simulink model "esp_env"  (R2020b)
settings: Solver=VariableStepAuto  StartTime=0.0  StopTime=7.1  RelTol=1e-3
values from neighbouring files (symbols this model uses):
  Ts = 1.0    (= 1)    [demo_rl.m]
undefined symbols (not defined in the file or in its folder): A, B, C, D, K, L, steeringAngle
libraries: simulink x2
settings Model: Creator=Shreyash  LastModifiedBy=Asus
settings DataIOCC: ReturnWorkspaceOutputs=off
settings DebuggingCC: ArithmeticOperatorsInVariantConditions=warning
settings SFSimCC: SimUseLocalCustomCode=off  CustomCodeUndefinedFunction=UseInterfaceOnly
settings RTWCC: RTWUseLocalCustomCode=off

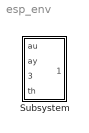
== system esp_env ==
  Subsystem : Subsystem

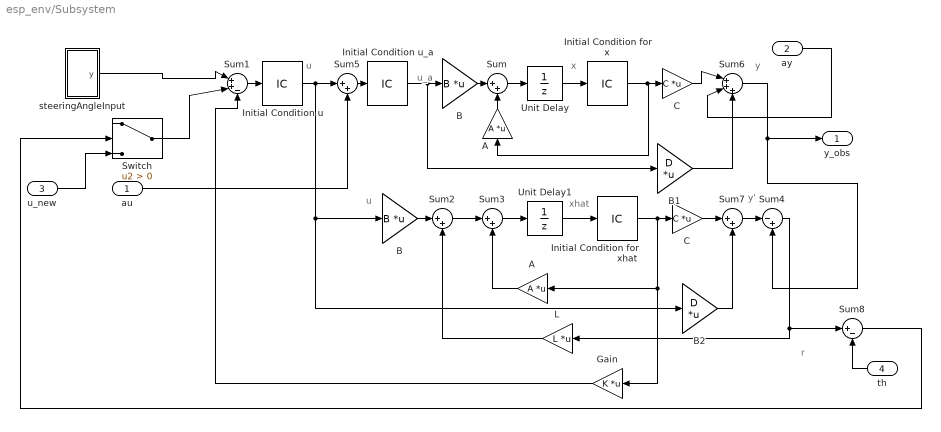
== system esp_env/Subsystem ==
  note: y
  note: r
  note: y'
  note: u
  note: u
  note: x
  note: xhat
  note: u_a
  au : Inport
  ay : Inport  Port=2
  u_new : Inport  Port=3
  th : Inport  Port=4
  A : Gain  Gain=A  Multiplication=Matrix(K*u)
  "A " : Gain  Gain=A  Multiplication=Matrix(K*u)
  B : Gain  Gain=B  Multiplication=Matrix(K*u)
  "B " : Gain  Gain=B  Multiplication=Matrix(K*u)
  B1 : Gain  Gain=D  Multiplication=Matrix(K*u)
  B2 : Gain  Gain=D  Multiplication=Matrix(K*u)
  C : Gain  Gain=C  Multiplication=Matrix(K*u)
  "C " : Gain  Gain=C  Multiplication=Matrix(K*u)
  Gain : Gain  Gain=K  Multiplication=Matrix(K*u)
  Initial Condition u : InitialCondition  Value=[0;0]
  "Initial Condition u_a " : InitialCondition  Value=[0;0]
  Initial Condition for x : InitialCondition  Value=[0;0]
  Initial Condition for xhat : InitialCondition  Value=[0;0]
  L : Gain  Gain=L  Multiplication=Matrix(K*u)
  Sum{,2..3,5,7} (5 alike) : Sum  Inputs=|++
  Sum1 : Sum  Inputs=|++-
  Sum4 : Sum  Inputs=|-+
  Sum6 : Sum  Inputs=|+++
  Sum8 : Sum  Inputs=|+-
  Switch : Switch  Criteria=u2 > Threshold
  Unit Delay : UnitDelay  SampleTime=-1  HasFrameUpgradeWarning=on
  Unit Delay1 : UnitDelay  SampleTime=-1  HasFrameUpgradeWarning=on
  steeringAngleInput : Subsystem
  y_obs : Outport
  wires:
  "A "/1 -> Sum/2
  Sum2/1 -> Sum3/1
  B1/1 -> Sum6/3
  L/1 -> Sum2/2
  Unit Delay/1 -> Initial Condition for x/1
  ay/1 -> Sum6/2
  Initial Condition for x/1 -> "C "/1, "A "/1
  Sum5/1 -> "Initial Condition u_a "/1
  Sum3/1 -> Unit Delay1/1
  Initial Condition for xhat/1 -> C/1, A/1, Gain/1
  Gain/1 -> Sum1/3
  "Initial Condition u_a "/1 -> B1/1, "B "/1
  Initial Condition u/1 -> B/1, B2/1, Sum5/1
  au/1 -> Sum5/2
  A/1 -> Sum3/2
  Sum/1 -> Unit Delay/1
  steeringAngleInput/1(y) -> Sum1/1
  Sum4/1 -> Sum8/1, L/1
  Sum1/1 -> Initial Condition u/1
  Unit Delay1/1 -> Initial Condition for xhat/1
  "C "/1 -> Sum6/1
  B/1 -> Sum2/1
  C/1 -> Sum7/1
  B2/1 -> Sum7/2
  u_new/1 -> Switch/3
  "B "/1 -> Sum/1
  Sum7/1 -> Sum4/1
  Sum6/1 -> y_obs/1, Sum4/2
  Switch/1 -> Sum1/2
  th/1 -> Sum8/2
  Sum8/1 -> Switch/2

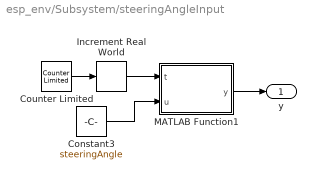
== system esp_env/Subsystem/steeringAngleInput ==
  Constant3 : Constant  Value=steeringAngle  SampleTime=Ts
  Counter Limited : simulink/Sources/Counter Limited  uplimit=size(steeringAngle,2)-1  tsamp=Ts
  Increment Real World : simulink/Additional Math & Discrete/Additional Math: Increment - Decrement/Increment Real World
      settings: SourceProductBaseCode=SL
  MATLAB Function1 : MATLAB Function  TreatAsAtomicUnit=on
  y : Outport
  wires:
  Counter Limited/1 -> Increment Real World/1
  Increment Real World/1 -> MATLAB Function1/1(t)
  MATLAB Function1/1(y) -> y/1
  Constant3/1 -> MATLAB Function1/2(u)

== matlab function esp_env/Subsystem/steeringAngleInput/MATLAB Function1 ==
  data: t input; u input; y output
function y = fcn(t, u)
y = u(t)*(pi/180)*0.0625;
%for t = 1 :100
    %y = au(:, t);
    %y = (-1 + 2.*rand(1, 2))'; 
end
